simulink model "dve_nadrze_linearized"  (R2020a)
settings: Solver=VariableStepAuto  StartTime=0.0  StopTime=t  RelTol=1e-3
values from neighbouring files (symbols this model uses):
  A = A_1    [control_file.m]
  B = B_1    [control_file.m]
  C = C_1    [control_file.m]
  D = D_1    [control_file.m]
  dQ = 0*U    (= 0)    [control_file.m]
  H1r = h1condition    (= 0)    [control_file.m]
  H2r = h2condition    (= 0)    [control_file.m]
  stepTime = t/4    (= 500)    [control_file.m]
  U = 1.2*i    [control_file.m]
settings Model: Creator=Filip Jašek  LastModifiedBy=Filip Jašek

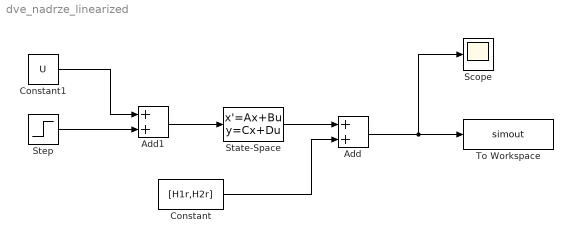
== system dve_nadrze_linearized ==
  Add : Sum
  Add1 : Sum
  Constant : Constant  Value=[H1r,H2r]
  Constant1 : Constant  Value=U
  Scope : Scope
  State-Space : StateSpace  A=A  B=B  C=C  D=D  InitialCondition=0
  Step : Step  Time=stepTime  After=dQ  SampleTime=0
  To Workspace : ToWorkspace  VariableName=simout  SaveFormat=Timeseries  SampleTime=-1
  wires:
  State-Space/1 -> Add/1
  Constant/1 -> Add/2
  Add/1 -> Scope/1, To Workspace/1
  Constant1/1 -> Add1/1
  Step/1 -> Add1/2
  Add1/1 -> State-Space/1
